simulink model "Non_Linear_Control_Paper_Graph_Recreation"  (R2018a)
settings: Solver=VariableStepAuto  StartTime=0.0  StopTime=16.0  RelTol=1e-3
settings Model: Creator=ASUS  LastModifiedBy=ASUS

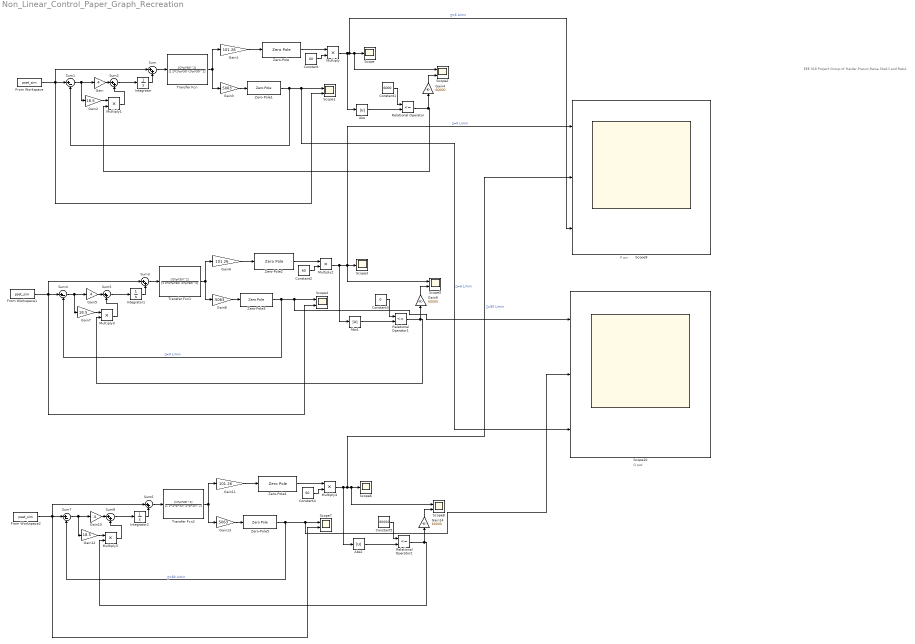
== system Non_Linear_Control_Paper_Graph_Recreation ==
  note: EEE 318 Project
      | Group of Haider,Prasun,Raisa
      | Shakil and Ratul.
  note: Q pat
  note: P aw
  Abs : Abs
  Abs1 : Abs
  Abs2 : Abs
  Constant : Constant  Value=60
  Constant1 : Constant  Value=6000
  Constant2 : Constant  Value=60
  Constant3 : Constant  Value=0
  Constant4 : Constant  Value=60
  Constant5 : Constant  Value=80000
  From Workspace : FromWorkspace  VariableName=pset_sim  SampleTime=0
  From Workspace1 : FromWorkspace  VariableName=pset_sim  SampleTime=0
  From Workspace2 : FromWorkspace  VariableName=pset_sim  SampleTime=0
  Gain : Gain  Gain=.4
  Gain1 : Gain  Gain=101.26
  Gain10 : Gain  Gain=.4
  Gain11 : Gain  Gain=101.26
  Gain12 : Gain  Gain=18.5
  Gain13 : Gain  Gain=.5063
  Gain14 : Gain  Gain=60000
  Gain2 : Gain  Gain=18.5
  Gain3 : Gain  Gain=.5063
  Gain4 : Gain  Gain=60000
  Gain5 : Gain  Gain=.4
  Gain6 : Gain  Gain=101.26
  Gain7 : Gain  Gain=18.5
  Gain8 : Gain  Gain=.5063
  Gain9 : Gain  Gain=60000
  Integrator : Integrator
  Integrator1 : Integrator
  Integrator2 : Integrator
  Multiply{,1..5} (6 alike) : Product
  Relational Operator : RelationalOperator  Operator=<=  OutDataTypeStr=boolean  RndMeth=Simplest
  Relational Operator1 : RelationalOperator  Operator=<=  OutDataTypeStr=boolean  RndMeth=Simplest
  Relational Operator2 : RelationalOperator  Operator=<=  OutDataTypeStr=boolean  RndMeth=Simplest
  Scope : Scope
  Scope{1..2,4..5,7..8} (6 alike) : Scope  NumInputPorts=2
  Scope10 : Scope  NumInputPorts=3
  Scope3 : Scope
  Scope6 : Scope
  Scope9 : Scope  NumInputPorts=3
  Sum{,2..3,5..6,8} (6 alike) : Sum  Inputs=|++
  Sum1 : Sum  Inputs=|+-
  Sum4 : Sum  Inputs=|+-
  Sum7 : Sum  Inputs=|+-
  Transfer Fcn : TransferFcn  Numerator=[(2*pi*30)^2]  Denominator=[1 2*(2*pi*30) (2*pi*30)^2]
  Transfer Fcn1 : TransferFcn  Numerator=[(2*pi*30)^2]  Denominator=[1 2*(2*pi*30) (2*pi*30)^2]
  Transfer Fcn2 : TransferFcn  Numerator=[(2*pi*30)^2]  Denominator=[1 2*(2*pi*30) (2*pi*30)^2]
  Zero-Pole : ZeroPole  Zeros=[-8.88e-16]  Poles=[-5.4436]
  Zero-Pole1 : ZeroPole  Zeros=[-10]  Poles=[-5.4436]
  Zero-Pole2 : ZeroPole  Zeros=[-8.88e-16]  Poles=[-5.4436]
  Zero-Pole3 : ZeroPole  Zeros=[-10]  Poles=[-5.4436]
  Zero-Pole4 : ZeroPole  Zeros=[-8.88e-16]  Poles=[-5.4436]
  Zero-Pole5 : ZeroPole  Zeros=[-10]  Poles=[-5.4436]
  wires:
  From Workspace/1 -> Scope1/2, Sum/1, Sum1/1
  Gain3/1 -> Zero-Pole1/1
  Constant/1 -> Multiply/2
  Sum1/1 -> Gain2/1, Gain/1
  Multiply/1 -> Abs/1, Scope9/3, Scope2/1, Scope/1  "𝛿=6 L/min"
  Gain1/1 -> Zero-Pole/1
  Transfer Fcn/1 -> Gain3/1, Gain1/1
  Integrator/1 -> Sum/2
  Sum/1 -> Transfer Fcn/1
  Zero-Pole1/1 -> Scope10/3, Scope1/1, Sum1/2  "𝛿=6 L/min"
  Zero-Pole/1 -> Multiply/1
  Constant1/1 -> Relational Operator/1
  Gain2/1 -> Multiply1/1
  Gain/1 -> Sum2/1
  Multiply1/1 -> Sum2/2
  Sum2/1 -> Integrator/1
  Relational Operator/1 -> Multiply1/2, Gain4/1
  Gain4/1 -> Scope2/2
  Abs/1 -> Relational Operator/2
  Transfer Fcn1/1 -> Gain8/1, Gain6/1
  Abs1/1 -> Relational Operator1/2
  From Workspace1/1 -> Scope4/2, Sum3/1, Sum4/1
  Relational Operator1/1 -> Multiply3/2, Gain9/1
  Constant3/1 -> Relational Operator1/1
  Sum5/1 -> Integrator1/1
  Gain5/1 -> Sum5/1
  Sum4/1 -> Gain7/1, Gain5/1
  Multiply3/1 -> Sum5/2
  Constant2/1 -> Multiply2/2
  Integrator1/1 -> Sum3/2
  Gain6/1 -> Zero-Pole2/1
  Sum3/1 -> Transfer Fcn1/1
  Zero-Pole3/1 -> Scope10/1, Scope4/1, Sum4/2  "𝛿=0 L/min"
  Gain9/1 -> Scope5/2
  Multiply2/1 -> Abs1/1, Scope9/1, Scope5/1, Scope3/1  "𝛿=0 L/min"
  Gain7/1 -> Multiply3/1
  Zero-Pole2/1 -> Multiply2/1
  Gain8/1 -> Zero-Pole3/1
  Transfer Fcn2/1 -> Gain13/1, Gain11/1
  Abs2/1 -> Relational Operator2/2
  From Workspace2/1 -> Scope7/2, Sum6/1, Sum7/1
  Relational Operator2/1 -> Multiply5/2, Gain14/1
  Constant5/1 -> Relational Operator2/1
  Sum8/1 -> Integrator2/1
  Gain10/1 -> Sum8/1
  Sum7/1 -> Gain12/1, Gain10/1
  Multiply5/1 -> Sum8/2
  Constant4/1 -> Multiply4/2
  Integrator2/1 -> Sum6/2
  Gain11/1 -> Zero-Pole4/1
  Sum6/1 -> Transfer Fcn2/1
  Zero-Pole5/1 -> Scope10/2, Scope7/1, Sum7/2  "𝛿=80 L/min"
  Gain14/1 -> Scope8/2
  Multiply4/1 -> Abs2/1, Scope9/2, Scope8/1, Scope6/1  "𝛿=80 L/min"
  Gain12/1 -> Multiply5/1
  Zero-Pole4/1 -> Multiply4/1
  Gain13/1 -> Zero-Pole5/1
